simulink model "Q1_half"  (R2018a)
settings: Solver=VariableStepAuto  StartTime=2  StopTime=5  RelTol=1e-3
libraries: powerlib x11, powerlib_meascontrol x1
settings Model: Creator=ROG  LastModifiedBy=furkan

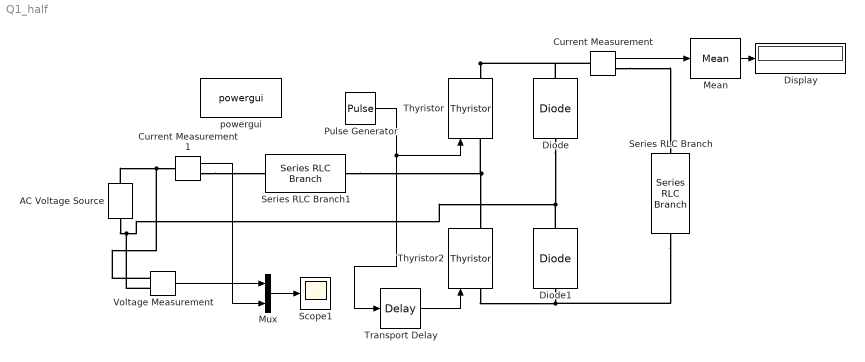
== system Q1_half ==
  AC Voltage Source : powerlib/Electrical Sources/AC Voltage Source  Amplitude=325  Phase=0  Frequency=50  SampleTime=0  Measurements=None  BusType=swing  Pref=10e3  Qref=0  Qmin=-inf  Qmax=+inf
  Current Measurement : powerlib/Measurements/Current Measurement  PhasorSimulation=off  OutputType=Complex  PSBequivalent=0
  Current Measurement1 : powerlib/Measurements/Current Measurement  PhasorSimulation=off  OutputType=Complex  PSBequivalent=0
  Diode : powerlib/Power Electronics/Diode  Ron=0.001  Lon=0  Vf=0  IC=0  UseSnubber=0  Rs=500  Cs=250e-9  Measurements=off
  Diode1 : powerlib/Power Electronics/Diode  Ron=0.001  Lon=0  Vf=0  IC=0  UseSnubber=0  Rs=500  Cs=250e-9  Measurements=off
  Display : Display
  Mean : powerlib_meascontrol/Measurements/Mean  Freq=60  Vinit=0  Ts=0
  Mux : Mux  Inputs=2
  Pulse Generator : DiscretePulseGenerator  PulseType=Time based  Amplitude=5  Period=0.02  PulseWidth=5  PhaseDelay=(57*0.02)/360
  Scope1 : Scope
  Series RLC Branch : powerlib/Elements/Series RLC Branch  LConnTagsString=__new0  RConnTagsString=__new0  BranchType=RL  Resistance=4  Inductance=0.2  SetiL0=off  InitialCurrent=0  Capacitance=1e-6  Setx0=off  InitialVoltage=0  Measurements=None
  Series RLC Branch1 : powerlib/Elements/Series RLC Branch  LConnTagsString=__new0  RConnTagsString=__new0  BranchType=L  Resistance=1  Inductance=0.5e-3  SetiL0=off  InitialCurrent=0  Capacitance=1e-6  Setx0=off  InitialVoltage=0  Measurements=None
  Thyristor : powerlib/Power Electronics/Thyristor  Ron=0.001  Lon=0  Vf=0  IC=0  Rs=500  Cs=250e-9  Measurements=on
  Thyristor2 : powerlib/Power Electronics/Thyristor  Ron=0.001  Lon=0  Vf=0  IC=0  Rs=500  Cs=250e-9  Measurements=on
  Transport Delay : TransportDelay  DelayTime=0.01
  Voltage Measurement : powerlib/Measurements/Voltage Measurement  PhasorSimulation=off  OutputType=Complex  PSBequivalent=0
  powergui : powerlib/powergui  Priority=1  SimulationMode=Discrete  SampleTime=5e-6  frequency=60  Iterations=50  frequencyindice=50  Pbase=100e6  ErrMax=1e-4  UnitsV=kV  UnitsW=MW  buscounter=0  FunctionMessages=off  echomessages=off  EnableUseOfTLC=off  CurrentSourceSwitches=off  DisableSnubberDevices=off  DisableRonSwitches=off  DisableVfSwitches=off  DisplayEquations=off  SolverType=Tustin/Backward Euler (TBE)  Interpol=off  ExternalGateDelay=off  methode=off  Ts=100  x0status=blocks  SPID=off  SwTol=0  HookPort=off  RestoreLinks=warning  ResistiveCurrentMeasurement=off  Frange=[0:2:500]  Ylog=off  Xlog=on  ShowGrid=off  save=off  variable=ZData  structure=InputCurrent  ZoomFFT=off  StartTime=2.5  cycles=100  DisplayStyle=2  fundamental=50  FreqAxis=off  MaxFrequency=1000  frequencyindicesteady=1  RmsSteady=1  display=off
  wires:
  Mean/1 -> Display/1
  Pulse Generator/1 -> Thyristor/1, Transport Delay/1
  Transport Delay/1 -> Thyristor2/1
  Voltage Measurement/1 -> Mux/1
  Current Measurement1/1 -> Mux/2
  Mux/1 -> Scope1/1
  Current Measurement/1 -> Mean/1
  connections:
  AC Voltage Source/RConn1 -- Voltage Measurement/LConn1 -- Current Measurement1/LConn1
  Current Measurement/RConn1 -- Series RLC Branch/LConn1
  Thyristor/RConn1 -- Current Measurement/LConn1 -- Diode/RConn1
  Series RLC Branch1/RConn1 -- Thyristor/LConn1 -- Thyristor2/RConn1
  AC Voltage Source/LConn1 -- Voltage Measurement/LConn2 -- Diode1/RConn1 -- Diode/LConn1
  Thyristor2/LConn1 -- Series RLC Branch/RConn1 -- Diode1/LConn1
  Current Measurement1/RConn1 -- Series RLC Branch1/LConn1
